simulink model "upControl"  (R2017b)
settings: Solver=FixedStepAuto  StartTime=0.0  StopTime=10.0  FixedStep=1e-3  RelTol=1e-9
values from neighbouring files (symbols this model uses):
  Khinf = designHinf(A2, B2, [0;1;0;0], Q, R, gamma)    [calcSystem.m]    (also in designHinf.m = inv(D21' * D21)*B22'*P)
settings Model: Creator=Haotian  LastModifiedBy=Haotian

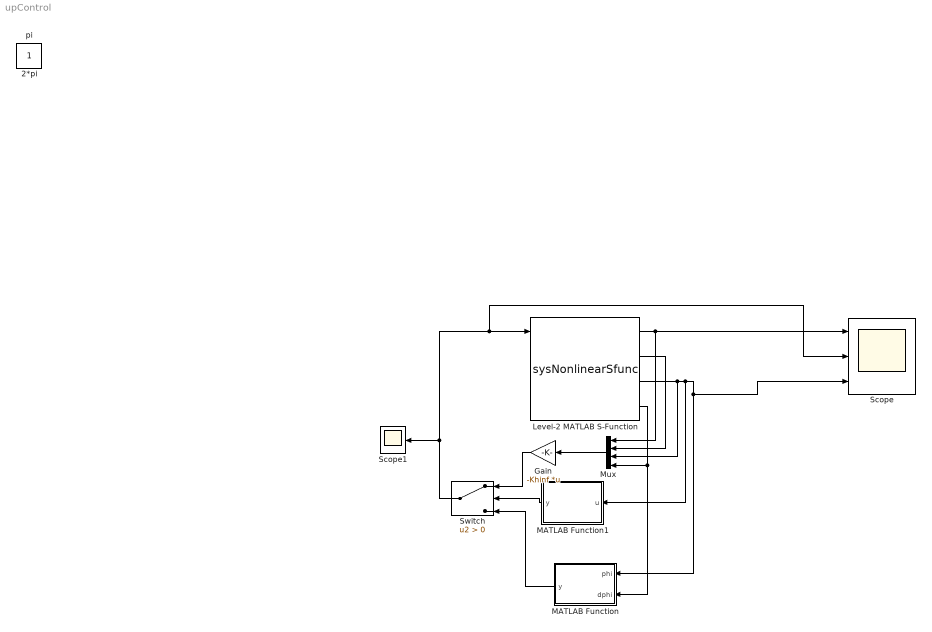
== system upControl ==
  Gain : Gain  Gain=-Khinf  Multiplication=Matrix(K*u)
  Level-2 MATLAB S-Function : M-S-Function  FunctionName=sysNonlinearSfunc  Parameters=Mc, Mg, b, l, I, init_phi, useAcc  mask(S-function: sysNonlinearSfunc){Mc=1.096, Mg=0.109, b=0.1, l=0.25, I=0.0034, init_phi=pi - 0.001, useAcc=on}
      mask prompts: Mc "小车质量"; Mg "摆杆质量"; b "小车摩擦系数"; l "摆杆转动轴心到杆质心的长度"; I "摆杆惯量"; init_phi "初始垂直夹角"; useAcc "使用加速度作为输入"
      mask help: 一阶倒立摆非线性模型。
      mask Display:
      | fprintf('一阶倒立摆\n\nM=%.3f m=%.3f\nb=%.3f l=%.3f\nI=%.3f phi0=%.2f', Mc, Mg, b, l, I, init_phi);
      | if(useAcc)
      |     port_label('input', 1, 'a');
      | else
      |     port_label('input', 1, 'F');
      | end
      | port_label('input', 2, 'ix');
      | port_label('input', 3, 'iv');
      | port_label('input', 4, 'i\phi','texmode','on');
      | 
      | port_label('output', 1, 'x');
      | port_label('output', 2, 'v');
      | port_label('output', 3, '\phi','texmode','on');
      | port_label('output', 4, 'd\phi','texmode','on');
  MATLAB Function : MATLAB Function  TreatAsAtomicUnit=on
  MATLAB Function1 : MATLAB Function  TreatAsAtomicUnit=on
  Mux : Mux
  Scope : Scope  NumInputPorts=3
  Scope1 : Scope
  Switch : Switch  Criteria=u2 > Threshold
  2*pi : Constant  IOType=siggen
  pi : Constant  IOType=siggen
  wires:
  Level-2 MATLAB S-Function/1 -> Mux/1, Scope/1
  Mux/1 -> Gain/1
  Level-2 MATLAB S-Function/4 -> MATLAB Function/2(dphi), Mux/4
  Level-2 MATLAB S-Function/2 -> Mux/2
  Gain/1 -> Switch/1
  Switch/1 -> Scope1/1, Scope/2, Level-2 MATLAB S-Function/1
  MATLAB Function/1(y) -> Switch/3
  MATLAB Function1/1(y) -> Switch/2
  Level-2 MATLAB S-Function/3 -> Mux/3, MATLAB Function1/1(u), Scope/3, MATLAB Function/1(phi)

== matlab function upControl/MATLAB Function1 ==
  data: u input; y output
function y = fcn(u)
if(abs(u) < pi/8)
    y = 1;
else
    y = 0;
end

== matlab function upControl/MATLAB Function ==
  data: phi input; y output; dphi input
function y = fcn(phi, dphi)
eps = 1e-3;
n = 0.15;
m = 0.109;
l = 0.25;
I = 0.0034;
g = 9.80;
if(abs(cos(phi)) < eps || abs(dphi) < eps)
   y = 0; 
else
y = -sign((1/2*I*dphi^2+m*g*l*(cos(phi)-1))*dphi*cos(phi)) * n * g;
end
